simulink model "Traslational_Motion_Observer"  (R2016b)
settings: Solver=VariableStepAuto  StartTime=0.0  StopTime=10.0  RelTol=1e-3
settings Model: Creator=liana  LastModifiedBy=liana

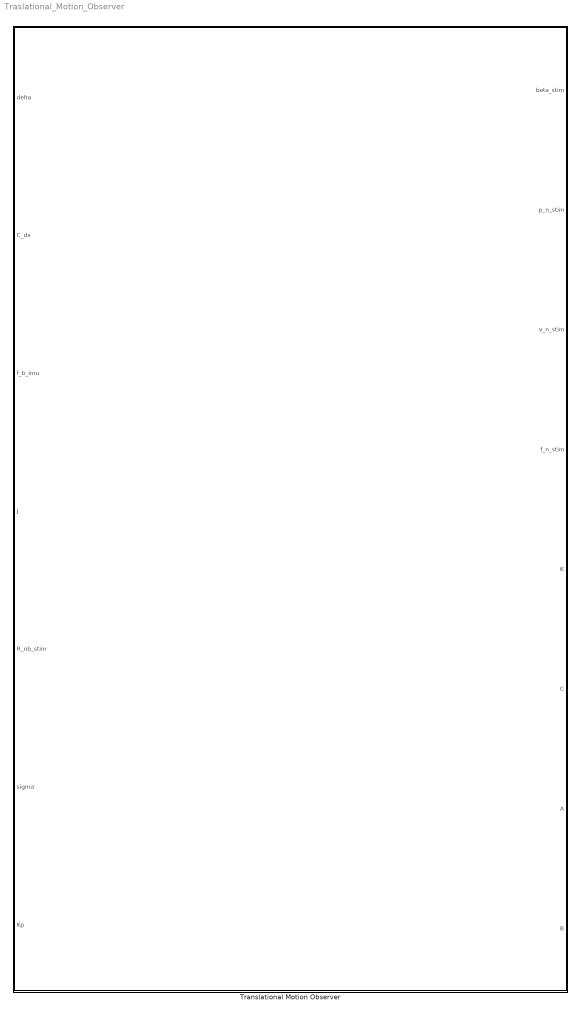
== system Traslational_Motion_Observer ==
  Translational Motion Observer : Subsystem

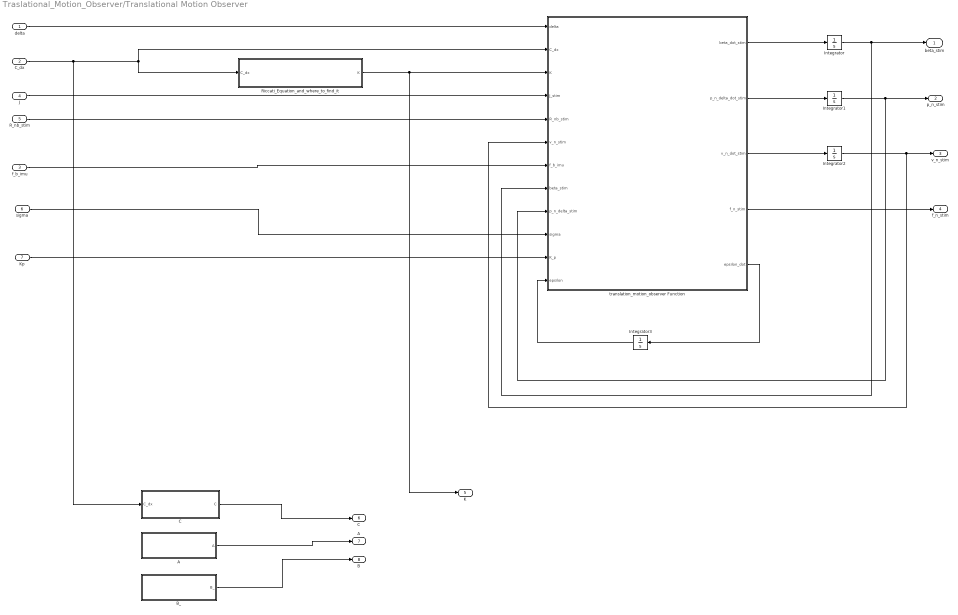
== system Traslational_Motion_Observer/Translational Motion Observer ==
  delta : Inport
  C_dx : Inport  Port=2
  f_b_imu : Inport  Port=3
  J : Inport  Port=4
  R_nb_stim : Inport  Port=5
  sigma : Inport  Port=6
  Kp : Inport  Port=7
  A : MATLAB Function  TreatAsAtomicUnit=on
  B_ : MATLAB Function  TreatAsAtomicUnit=on
  C : MATLAB Function  TreatAsAtomicUnit=on
  Integrator{,1..3} (4 alike) : Integrator
  Riccati_Equation_and_where_to_find_it : Subsystem
  translation_motion_observer Function : MATLAB Function  TreatAsAtomicUnit=on
  beta_stim : Outport
  p_n_stim : Outport  Port=2
  v_n_stim : Outport  Port=3
  f_n_stim : Outport  Port=4
  K : Outport  Port=5
  "C " : Outport  Port=6
  " A" : Outport  Port=7
  B : Outport  Port=8
  wires:
  translation_motion_observer Function/4(f_n_stim) -> f_n_stim/1
  translation_motion_observer Function/3(v_n_dot_stim) -> Integrator2/1
  Integrator2/1 -> translation_motion_observer Function/6(v_n_stim), v_n_stim/1
  translation_motion_observer Function/2(p_n_delta_dot_stim) -> Integrator1/1
  Integrator1/1 -> translation_motion_observer Function/9(p_n_delta_stim), p_n_stim/1
  Integrator/1 -> translation_motion_observer Function/8(beta_stim), beta_stim/1
  translation_motion_observer Function/1(beta_dot_stim) -> Integrator/1
  translation_motion_observer Function/5(epsilon_dot) -> Integrator3/1
  Integrator3/1 -> translation_motion_observer Function/12(epsilon)
  C_dx/1 -> C/1(C_dx), translation_motion_observer Function/2(C_dx), Riccati_Equation_and_where_to_find_it/1(C_dx)
  J/1 -> translation_motion_observer Function/4(J_stim)
  R_nb_stim/1 -> translation_motion_observer Function/5(R_nb_stim)
  delta/1 -> translation_motion_observer Function/1(delta)
  f_b_imu/1 -> translation_motion_observer Function/7(f_b_imu)
  sigma/1 -> translation_motion_observer Function/10(sigma)
  Kp/1 -> translation_motion_observer Function/11(K_p)
  A/1(A) -> " A"/1
  C/1(C) -> "C "/1
  Riccati_Equation_and_where_to_find_it/1(K) -> K/1, translation_motion_observer Function/3(K)
  B_/1(B_) -> B/1

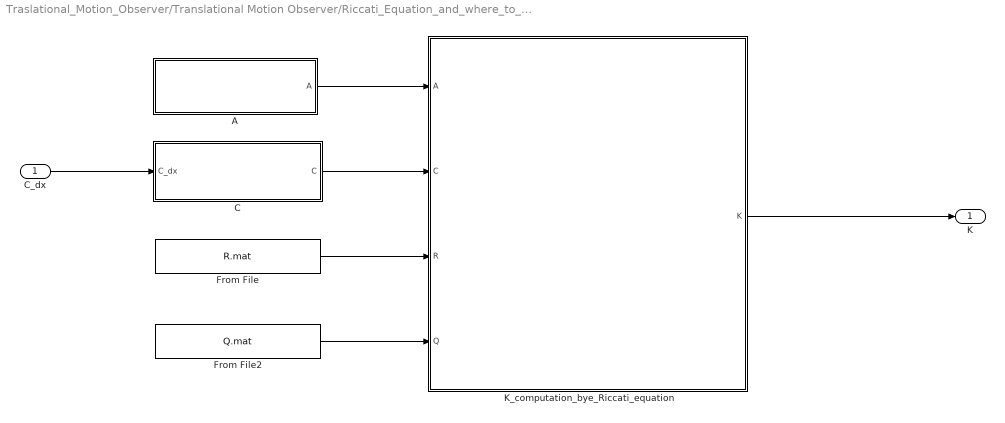
== system Traslational_Motion_Observer/Translational Motion Observer/Riccati_Equation_and_where_to_find_it ==
  C_dx : Inport
  A : MATLAB Function  TreatAsAtomicUnit=on
  C : MATLAB Function  TreatAsAtomicUnit=on
  From File : FromFile  FileName=R.mat  SampleTime=0
  From File2 : FromFile  FileName=Q.mat  SampleTime=0
  K_computation_bye_Riccati_equation : MATLAB Function  TreatAsAtomicUnit=on
  K : Outport
  wires:
  C_dx/1 -> C/1(C_dx)
  K_computation_bye_Riccati_equation/1(K) -> K/1
  From File/1 -> K_computation_bye_Riccati_equation/3(R)
  A/1(A) -> K_computation_bye_Riccati_equation/1(A)
  From File2/1 -> K_computation_bye_Riccati_equation/4(Q)
  C/1(C) -> K_computation_bye_Riccati_equation/2(C)

== matlab function Traslational_Motion_Observer/Translational Motion Observer/translation_motion_observer Function ==
  data: delta input; C_dx input; K input; beta_dot_stim output; J_stim input; R_nb_stim input; p_n_delta_dot_stim output; v_n_dot_stim output; f_n_stim output; v_n_stim input; f_b_imu input; beta_stim input; p_n_delta_stim input; sigma input; K_p input; epsilon_dot output; epsilon input
function [beta_dot_stim,p_n_delta_dot_stim,v_n_dot_stim,f_n_stim,epsilon_dot] =  TMO_func(delta,C_dx,K,J_stim,R_nb_stim, v_n_stim,f_b_imu, beta_stim, p_n_delta_stim,sigma,K_p,epsilon)

 K_pp = K(1:3,:); 
 K_beta_p = K(4,:);
 K_v_p = K(5:7,:);
 K_eps_p = K(8:10,:);
 %obtained by Riccati equation..


% remember to insert a clock to define dimensions of all variables

g_n = [0 0 1]';

x_stim = [p_n_delta_stim beta_stim];
delta_stim = 2*C_dx*x_stim;
delta_diff = (delta - delta_stim);



p_n_delta_dot_stim = v_n_stim + K_pp * delta_diff;        % eq 14


beta_dot_stim = K_beta_p * delta_diff;                       % eq 15


%theoretically we can't know epsilon
f_n_stim = R_nb_stim*f_b_imu + epsilon ;         % eq 18


v_n_dot_stim  = f_n_stim + g_n + K_v_p*delta_diff;         % eq 16


epsilon_dot   = -sigma*K_p*J_stim*f_b_imu + K_eps_p*delta_diff; % eq 17
end

== matlab function Traslational_Motion_Observer/Translational Motion Observer/Riccati_Equation_and_where_to_find_it/K_computation_bye_Riccati_equation ==
  data: A input; K output; C input; R input; Q input
function K = K_func(A,C,R,Q)

K = zeros(10,3);

coder.extrinsic('care');

[P,L,G] = care(A,C',Q,R);

R_inv = pinv(R); 

K = P*C'*R_inv;

== matlab function Traslational_Motion_Observer/Translational Motion Observer/Riccati_Equation_and_where_to_find_it/A ==
  data: A output
function A = A()

 A = zeros(10);

 A(1:3,5:7) = eye(3);
 A(5:7,8:10) = eye(3);
 
A;

== matlab function Traslational_Motion_Observer/Translational Motion Observer/Riccati_Equation_and_where_to_find_it/C ==
  data: C output; C_dx input
function C = C(C_dx)

   row = size(C_dx,1); 

   C1 = zeros(row,6);

 C = [2*C_dx C1];

== matlab function Traslational_Motion_Observer/Translational Motion Observer/A ==
  data: A output
function A = A()

 A = zeros(10);

 A(1:3,5:7) = eye(3);
 A(5:7,8:10) = eye(3);
 
end

== matlab function Traslational_Motion_Observer/Translational Motion Observer/C ==
  data: C output; C_dx input
function C = C(C_dx)

   row = size(C_dx,1); 

   C1 = zeros(row,6);

 C = [2*C_dx C1];
 
 
end

== matlab function Traslational_Motion_Observer/Translational Motion Observer/B_ ==
  data: B_ output
function B_ = B()

 B_ = zeros(10,3);

 B_(8:10,1:3) = eye(3);
end
